simulink model "Fast_CurrentWithoutSim"  (R2022b)
settings: Solver=VariableStepAuto  StartTime=0.0  StopTime=20  RelTol=1e-3
PreLoadFcn:
  | openManipulatorParameters;
  | 
  | % % Set sampling time for Simulink pace execution
  | % Ts = 0.005;
  | %
  | % % Set COM port
  | % com_port = 'COM6';
  | %
  | % % Set baudrate
  | % baud_rate = 1000000;
  | %
  | % % Set protocol Version
  | % protocol_version = 2;
  | %
  | % % Initialize library and port number
  | % [lib_name, port_num] = initDxl(com_port);
  | %
  | % % Open port
  | % openPortDxl(lib_name, port_num);
  | %
  | % % Set Baudrate
  | % setBaudDxl(lib_name, port_num, baud_rate);
  | %
  | % % Find dynamixels
  | % [motor_IDs, motor_models] = findDxl(lib_name, port_num, protocol_version);
  | %
  | % % Operating modes
  | % operatingModeDxl(lib_name, port_num, protocol_version, motor_IDs, ...
  | %     motor_models, 'Current Control');
  | %
  | % % Drive modes
  | % driveModeDxl(lib_name, port_num, protocol_version, motor_IDs, ...
  | %     motor_models, 'Time-based Profile');
  | %
  | % % Indirect addresses are accessible only when the torque is disabled
  | % torqueDxl(lib_name, port_num, protocol_version, motor_IDs, ...
  | %     motor_models, 'Disable');
  | %
  | % % Define the read and write quantities
  | % select_sync_write = "Goal Current";
  | % select_sync_read = "Present Position";
  | %
  | % % Set indirect addresses for fast sync write
  | % [start_address_write_indirect, data_length_write_indirect] = ...
  | %     setIndirectWriteDxl(lib_name, port_num, protocol_version, motor_IDs, ...
  | %     motor_models, select_sync_write);
  | %
  | % % Set indirect addresses for fast sync read
  | % start_address_read_indirect = start_address_write_indirect + ...
  | %     data_length_write_indirect;
  | % [start_address_read_indirect, data_length_read_indirect] = ...
  | %     setIndirectReadDxl(lib_name, port_num, protocol_version, motor_IDs, ...
  | %     motor_models, start_address_read_indirect, select_sync_read);
  | %
  | % % Enable torque
  | % torqueDxl(lib_name, port_num, protocol_version, motor_IDs, motor_models, ...
  | %     'Enable');
  | % % Check error
  | % checkErrorDxl(lib_name, port_num, protocol_version)
  | %
  | % % Initialize sync write
  | % group_num_write = initSyncWriteIndirectDxl(lib_name, port_num, protocol_version,...
  | %     motor_models, start_address_write_indirect, data_length_write_indirect);
  | %
  | % % Initialize sync read
  | % group_num_read = initSyncReadIndirectDxl(lib_name, port_num, protocol_version,...
  | %     motor_models, start_address_read_indirect, data_length_read_indirect);
  | %
  | % % Add parameters for the sync read
  | % syncReadAddParamDxl(lib_name, group_num_read, motor_IDs);
PostLoadFcn:
  | % % Read clear parameters
  | % syncReadClearParamDxl(lib_name, group_num_read);
  | %
  | % % Disable torque
  | % torqueDxl(lib_name, port_num, protocol_version, motor_IDs, motor_models, ...
  | %     'Disable');
  | %
  | % % Check error
  | % checkErrorDxl(lib_name, port_num, protocol_version)
  | %
  | % % Close port
  | % closePortDxl(lib_name,port_num);
StartFcn:
  | % % Set sampling time for Simulink pace execution
  | % Ts = 0.005;
  | %
  | % % Set COM port
  | % com_port = 'COM6';
  | %
  | % % Set baudrate
  | % baud_rate = 1000000;
  | %
  | % % Set protocol Version
  | % protocol_version = 2;
  | %
  | % % Initialize library and port number
  | % [lib_name, port_num] = initDxl(com_port);
  | %
  | % % Open port
  | % openPortDxl(lib_name, port_num);
  | %
  | % % Set Baudrate
  | % setBaudDxl(lib_name, port_num, baud_rate);
  | %
  | % % Find dynamixels
  | % [motor_IDs, motor_models] = findDxl(lib_name, port_num, protocol_version);
  | %
  | % % Operating modes
  | % operatingModeDxl(lib_name, port_num, protocol_version, motor_IDs, ...
  | %     motor_models, 'Current Control');
  | %
  | % % Drive modes
  | % driveModeDxl(lib_name, port_num, protocol_version, motor_IDs, ...
  | %     motor_models, 'Time-based Profile');
  | %
  | % % Indirect addresses are accessible only when the torque is disabled
  | % torqueDxl(lib_name, port_num, protocol_version, motor_IDs, ...
  | %     motor_models, 'Disable');
  | %
  | % % Define the read and write quantities
  | % select_sync_write = "Goal Current";
  | % select_sync_read = "Present Position";
  | %
  | % % Set indirect addresses for fast sync write
  | % [start_address_write_indirect, data_length_write_indirect] = ...
  | %     setIndirectWriteDxl(lib_name, port_num, protocol_version, motor_IDs, ...
  | %     motor_models, select_sync_write);
  | %
  | % % Set indirect addresses for fast sync read
  | % start_address_read_indirect = start_address_write_indirect + ...
  | %     data_length_write_indirect;
  | % [start_address_read_indirect, data_length_read_indirect] = ...
  | %     setIndirectReadDxl(lib_name, port_num, protocol_version, motor_IDs, ...
  | %     motor_models, start_address_read_indirect, select_sync_read);
  | %
  | % % Enable torque
  | % torqueDxl(lib_name, port_num, protocol_version, motor_IDs, motor_models, ...
  | %     'Enable');
  | % % Check error
  | % checkErrorDxl(lib_name, port_num, protocol_version)
  | %
  | % % Initialize sync write
  | % group_num_write = initSyncWriteIndirectDxl(lib_name, port_num, protocol_version,...
  | %     motor_models, start_address_write_indirect, data_length_write_indirect);
  | %
  | % % Initialize sync read
  | % group_num_read = initSyncReadIndirectDxl(lib_name, port_num, protocol_version,...
  | %     motor_models, start_address_read_indirect, data_length_read_indirect);
  | %
  | % % Add parameters for the sync read
  | % syncReadAddParamDxl(lib_name, group_num_read, motor_IDs);
StopFcn:
  | % % Read clear parameters
  | % syncReadClearParamDxl(lib_name, group_num_read);
  | %
  | % % Disable torque
  | % torqueDxl(lib_name, port_num, protocol_version, motor_IDs, motor_models, ...
  | %     'Disable');
  | %
  | % % Check error
  | % checkErrorDxl(lib_name, port_num, protocol_version)
  | %
  | % % Close port
  | % closePortDxl(lib_name,port_num);
undefined symbols (not defined in the file): Ts, TsCtrl
libraries: dxlSimLibrary x2, slDxl_lib x2, OpenManipulatorLib x1
settings Model: SimulationMode=accelerator  Creator=scastro  LastModifiedBy=Boog
settings SolverCC: AlgebraicLoopSolver=TrustRegion  DecoupledContinuousIntegration=on  MinimalZcImpactIntegration=on
settings DataIOCC: ReturnWorkspaceOutputs=off
settings DebuggingCC: ParameterOverflowMsg=none  UnconnectedInputMsg=warning  UnconnectedOutputMsg=warning  UnconnectedLineMsg=warning  SFMachineParentedDataDiag=warning  ArithmeticOperatorsInVariantConditions=warning
settings ModelReferenceCC: EnableRefExpFcnMdlSchedulingChecks=on
settings SFSimCC: SimUseLocalCustomCode=off  CustomCodeUndefinedFunction=UseInterfaceOnly
settings RTWCC: RTWUseLocalCustomCode=off
settings ExplorerConfigSet: InternalSimMechanicsExplorerSettings="<ExplorerConfiguration><canonicalview>default</canonicalview><AnimationSetting><BasePlaybackSpeed>1.0</BasePlaybackSpeed><PlaybackSpeedFactor>1.0</PlaybackSpeedFactor></AnimationSetting><TilePanel><TileInfo><Tiles Columns=\"1\" Count=\"1\" Rows=\"1\"><Column Weight=\"1\"/><Row Weight=\"1\"/><Tile Height=\"1\" Width=\"1\" X=\"0\" Y=\"0\"/></Tiles></TileInfo><SceneInfo><SceneViewer><BGColor><R>0.60000002384185791</R><G>0.60000002384185791</G><B>0.60000002384185791</B></BGColor><Camera><DoPerspective>off</DoPerspective><Position><X>0.428752942017998073</X><Y>-0.712150369953937545</Y><Z>0.628314823463847372</Z></Position><Center><X>0.0455703138120887447</X><Y>0.0802507835591396851</Y><Z>0.153687090021758288</Z></Center><Up><X>-0.128866037345358619</X><Y>0.462960972240881619</Y><Z>0.876961049648547597</Z></Up><ViewLimDist>1</ViewLimDist><YLim>0.579070269035580121</YLim><XLim>0.64437894599448009</XLim></Camera></SceneViewer></SceneInfo></TilePanel><MechEditorPanel><Cameras/><GfxPanelCameraMap/><VideoCreator><PlaybackSpeedRatio>1.0</PlaybackSpeedRatio><FrameRate>30</FrameRate><VideoFormat>Motion JPEG AVI</VideoFormat><FrameSize>auto</FrameSize></VideoCreator></MechEditorPanel></ExplorerConfiguration>"

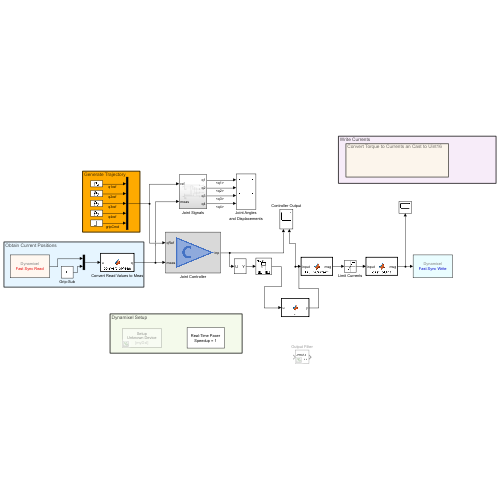
[thumbnail: Simulink's stored preview of the top-level diagram]
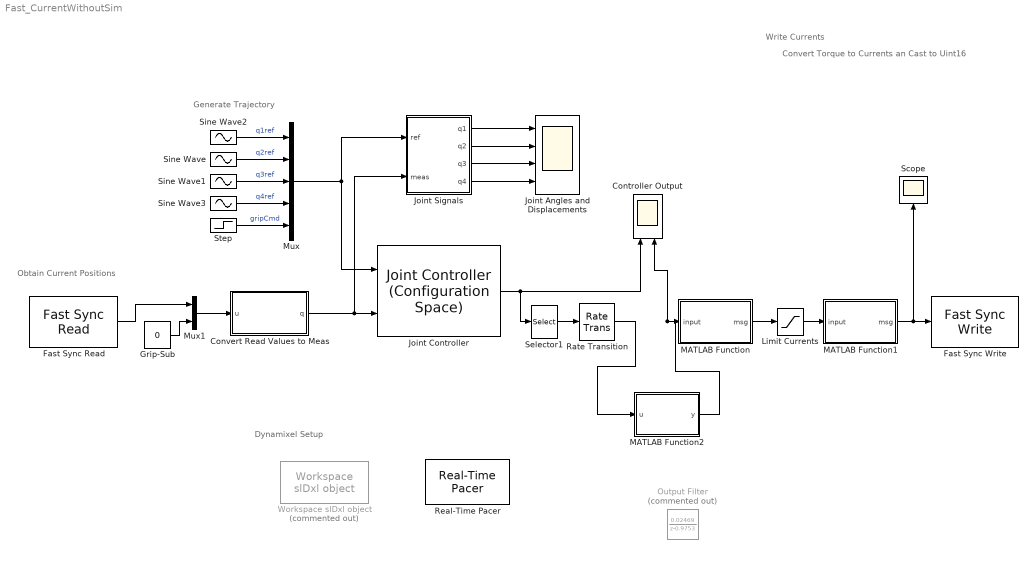
== system Fast_CurrentWithoutSim ==
  note: Dynamixel Setup
  note: Obtain Current Positions
  note: Generate Trajectory
  note: Write Currents
  note: Convert Torque to Currents an Cast to Uint16
  Controller Output : Scope  NumInputPorts=2
  Convert Read Values to Meas : MATLAB Function  TreatAsAtomicUnit=on
  Fast Sync Read : dxlSimLibrary/Fast Sync Read  Description=|  lib_name=lib_name  group_num_read=group_num_read  ids=motor_IDs  models=motor_models  select_sync_read=select_sync_read  start_address_read_indirect=start_address_read_indirect  Ts=Ts
      | Dynamixel library for Matlab and Simulink
      | Fast Sync Read function
      | Author: Georgios Andrikopoulos (geoand@kth.se), 2022 
      | Mechatronics & Embedded Control Systems Unit, KTH, Stockholm
  Fast Sync Write : dxlSimLibrary/Fast Sync Write  Description=|  lib_name=lib_name  group_num_write=group_num_write  ids=motor_IDs  models=motor_models  select_sync_write=select_sync_write  Ts=Ts
      | Dynamixel library for Matlab and Simulink
      | Fast Sync Write function
      | Author: Georgios Andrikopoulos (geoand@kth.se), 2022 
      | Mechatronics & Embedded Control Systems Unit, KTH, Stockholm
  Grip-Sub : Constant  Value=0
  Joint Angles and Displacements : Scope  NumInputPorts=4
  Joint Controller : OpenManipulatorLib/Joint Controller (Configuration Space)  SystemSampleTime=-1  VariantControl=ctrlType==1  VariantActivationTime=update diagram  Latency=0  AutoFrameSizeCalculation=off
      link override Saturate Inputs/Saturate  Joint Torques: UpperLimit=ctrlUpperLimit  LowerLimit=ctrlLowerLimit
  Joint Signals : Subsystem
  Limit Currents : Saturate  UpperLimit=200  LowerLimit=-200  OutDataTypeStr=int16
  MATLAB Function : MATLAB Function  TreatAsAtomicUnit=on
  MATLAB Function1 : MATLAB Function  TreatAsAtomicUnit=on
  MATLAB Function2 : MATLAB Function  TreatAsAtomicUnit=on
  Mux : Mux  Inputs=5
  Mux1 : Mux  Inputs=2
  Output Filter : DiscreteTransferFcn  Commented=on  Numerator=0.02469  Denominator=[1 -0.9753]
  Rate Transition : RateTransition
  Real-Time Pacer : slDxl_lib/Real-Time Pacer  simTimePerRealTime=1
  Scope : Scope
  Selector1 : Selector  InputPortWidth=6  IndexOptions=Index vector (dialog)  Indices=[1:5]  OutputSizes=1
  Sine Wave : Sin  Amplitude=-pi/6  Frequency=0.2  SampleTime=TsCtrl
  Sine Wave1 : Sin  Amplitude=-pi/6  Frequency=0.3  SampleTime=TsCtrl
  Sine Wave2 : Sin  Amplitude=2*pi/3  Frequency=.3  SampleTime=TsCtrl
  Sine Wave3 : Sin  Amplitude=pi/6  Frequency=0.25  SampleTime=TsCtrl
  Step : Step  Time=5  SampleTime=TsCtrl
  Workspace slDxl object : slDxl_lib/Workspace slDxl object  Commented=on  slDxlVarName=Existing Object Handle #1  workspaceVarName=myDxl
  wires:
  Sine Wave/1 -> Mux/2  "q2ref"
  Sine Wave1/1 -> Mux/3  "q3ref"
  Sine Wave2/1 -> Mux/1  "q1ref"
  Mux/1 -> Joint Controller/1, Joint Signals/1(ref)
  Joint Signals/1(q1) -> Joint Angles and Displacements/1
  Joint Signals/2(q2) -> Joint Angles and Displacements/2
  Joint Signals/3(q3) -> Joint Angles and Displacements/3
  Joint Signals/4(q4) -> Joint Angles and Displacements/4
  Sine Wave3/1 -> Mux/4  "q4ref"
  Step/1 -> Mux/5  "gripCmd"
  Joint Controller/1 -> Selector1/1, Controller Output/1
  Convert Read Values to Meas/1(q) -> Joint Controller/2, Joint Signals/2(meas)
  MATLAB Function/1(msg) -> Limit Currents/1
  Fast Sync Read/1 -> Mux1/1
  Mux1/1 -> Convert Read Values to Meas/1(u)
  Grip-Sub/1 -> Mux1/2
  Selector1/1 -> Rate Transition/1
  MATLAB Function1/1(msg) -> Fast Sync Write/1, Scope/1
  Limit Currents/1 -> MATLAB Function1/1(input)
  Rate Transition/1 -> MATLAB Function2/1(u)
  MATLAB Function2/1(y) -> Controller Output/2, MATLAB Function/1(input)

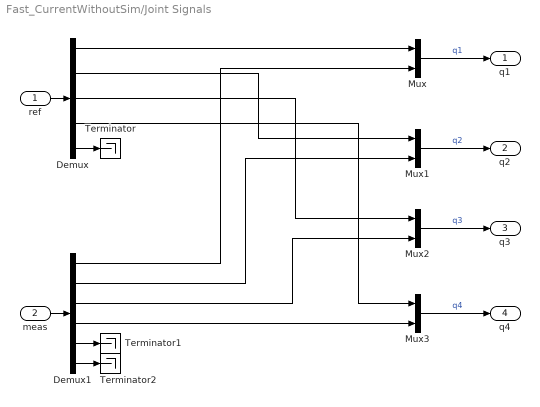
== system Fast_CurrentWithoutSim/Joint Signals ==
  ref : Inport
  meas : Inport  Port=2
  Demux : Demux  Outputs=5
  Demux1 : Demux  Outputs=6
  Mux{,1..3} (4 alike) : Mux  Inputs=2
  Terminator : Terminator
  Terminator1 : Terminator
  Terminator2 : Terminator
  q1 : Outport  VectorParamsAs1DForOutWhenUnconnected=off
  q2 : Outport  Port=2  VectorParamsAs1DForOutWhenUnconnected=off
  q3 : Outport  Port=3  VectorParamsAs1DForOutWhenUnconnected=off
  q4 : Outport  Port=4  VectorParamsAs1DForOutWhenUnconnected=off
  wires:
  Mux2/1 -> q3/1  "q3"
  ref/1 -> Demux/1
  Mux3/1 -> q4/1  "q4"
  Mux/1 -> q1/1  "q1"
  meas/1 -> Demux1/1
  Demux/1 -> Mux/1
  Demux1/1 -> Mux/2
  Mux1/1 -> q2/1  "q2"
  Demux/2 -> Mux1/1
  Demux1/2 -> Mux1/2
  Demux/3 -> Mux2/1
  Demux1/3 -> Mux2/2
  Demux1/4 -> Mux3/2
  Demux/4 -> Mux3/1
  Demux/5 -> Terminator/1
  Demux1/5 -> Terminator1/1
  Demux1/6 -> Terminator2/1

== matlab function Fast_CurrentWithoutSim/MATLAB Function ==
  data: input input; msg output
function msg = tauToCurrent(input)
    current_A = 0.5714 .* input;
    msg = current_A .* 1000 ./ 2.69;

== matlab function Fast_CurrentWithoutSim/Convert Read Values to Meas ==
  data: u input; q output
function q = convertToMeas(u)
% 3.14 / 2048
q = (0.001534355386369.*u) - 3.14;

== matlab function Fast_CurrentWithoutSim/MATLAB Function2 ==
  data: u input; y output
function y = fcn(u)

y = smoothdata(u);

== matlab function Fast_CurrentWithoutSim/MATLAB Function1 ==
  data: input input; msg output
function msg = castToUint(input)
    msg = zeros(size(input));
    for i = 1:length(input)
        msg(i) = typecast(int16(input(i)), "uint16");
    end
end
